simulink model "BP_PID"  (R2019b)
settings: Solver=FixedStepAuto  StartTime=0.0  StopTime=500  FixedStep=0.01  RelTol=1e-3  EnableMultiTasking=on
settings Model: Creator=Becca  LastModifiedBy=lenovo
settings DataIOCC: ReturnWorkspaceOutputs=off
settings OptimizationCC: LifeSpan=inf
settings DebuggingCC: SFUnexpectedBacktrackingDiag=warning  SFNoUnconditionalDefaultTransitionDiag=warning  ArithmeticOperatorsInVariantConditions=warning
settings SFSimCC: SimUseLocalCustomCode=off  CustomCodeUndefinedFunction=UseInterfaceOnly
settings RTWCC: RTWUseLocalCustomCode=off
settings CodeAppCC: StateflowObjectComments=on
settings GRTTargetCC: TargetLangStandard=C89/C90 (ANSI)  GeneratePreprocessorConditionals=Disable all
settings ConfigComp: CovMetricSettings=dw  CovHtmlReporting=on  CovSaveCumulativeToWorkspaceVar=on  CovSaveSingleToWorkspaceVar=on  CovExternalEMLEnable=off

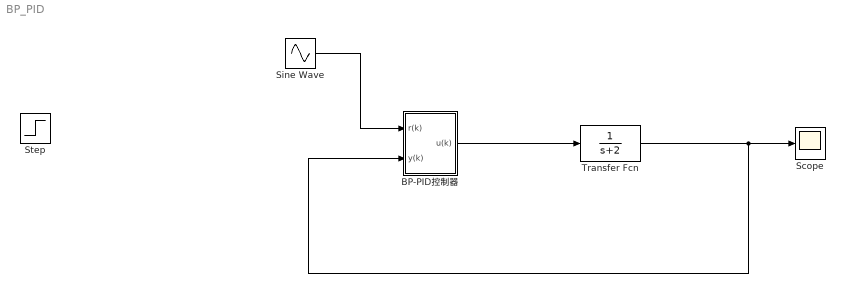
== system BP_PID ==
  BP-PID控制器 : Subsystem
  Scope : Scope
  Sine Wave : Sin  Frequency=2  SampleTime=0
  Step : Step  SampleTime=0
  Transfer Fcn : TransferFcn  Denominator="[1  2]"
  wires:
  Transfer Fcn/1 -> BP-PID控制器/2(y(k)), Scope/1
  BP-PID控制器/1(u(k)) -> Transfer Fcn/1
  Sine Wave/1 -> BP-PID控制器/1(r(k))

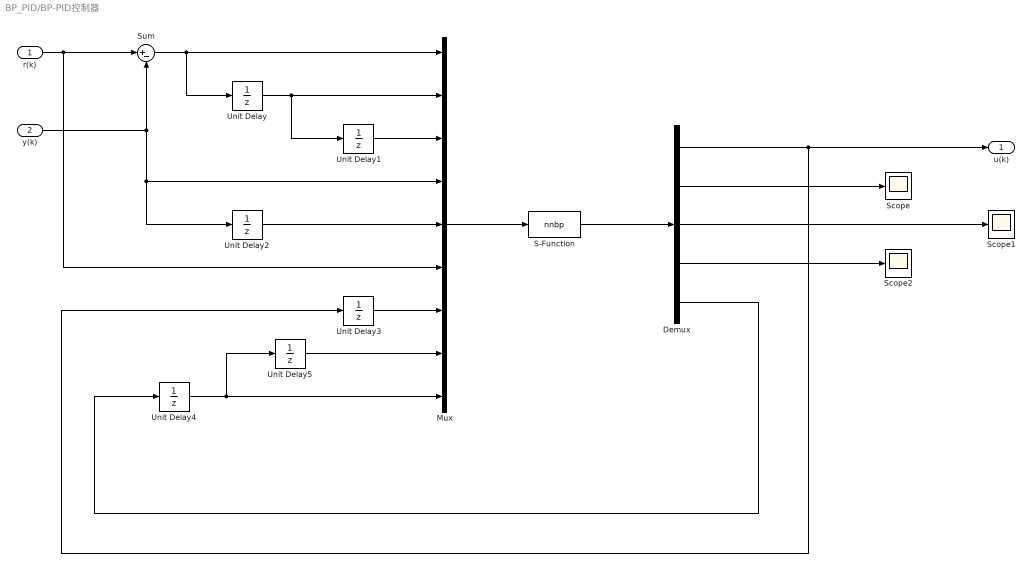
== system BP_PID/BP-PID控制器 ==
  r(k) : Inport
  y(k) : Inport  Port=2
  Demux : Demux  Outputs=[1 1 1 1 48]
  Mux : Mux  Inputs=9
  S-Function : S-Function  FunctionName=nnbp  Parameters=T,nh,xite,alfa  SFunctionDeploymentMode=off  EnableBusSupport=off  mask{T=0.01, nh=8, xite=0.3, alfa=0.3}
  Scope : Scope
  Scope1 : Scope
  Scope2 : Scope
  Sum : Sum  Inputs=|+-
  Unit Delay{,1..5} (6 alike) : UnitDelay  SampleTime=-1  HasFrameUpgradeWarning=on
  u(k) : Outport
  wires:
  r(k)/1 -> Sum/1, Mux/6
  y(k)/1 -> Sum/2, Unit Delay2/1, Mux/4
  Sum/1 -> Unit Delay/1, Mux/1
  Unit Delay/1 -> Unit Delay1/1, Mux/2
  Unit Delay1/1 -> Mux/3
  Unit Delay2/1 -> Mux/5
  Mux/1 -> S-Function/1
  Unit Delay3/1 -> Mux/7
  Unit Delay5/1 -> Mux/8
  Unit Delay4/1 -> Unit Delay5/1, Mux/9
  S-Function/1 -> Demux/1
  Demux/1 -> Unit Delay3/1, u(k)/1
  Demux/2 -> Scope/1
  Demux/3 -> Scope1/1
  Demux/4 -> Scope2/1
  Demux/5 -> Unit Delay4/1
